simulink model "SVC"  (R2015b)
settings: Solver=VariableStepAuto  StartTime=0.0  StopTime=3  MaxStep=Ts  RelTol=1e-3
values from neighbouring files (symbols this model uses):
  f = 50    [ThreePhaseVSC_Code.m]
  FC_C = TSC_C    (= 3.3135e-06)    [ThreePhaseVSC_Code.m]
  FC_L = 122.3114e-3    (= 0.1223114)    [ThreePhaseVSC_Code.m]
  FC_R = 10    [ThreePhaseVSC_Code.m]
  L = XL/(2*2*pi*f)    (= 0.159154943092)    [ThreePhaseVSC_Code.m]
  TCR_L = 517.59e-3    (= 0.51759)    [ThreePhaseVSC_Code.m]
  TCR_R = 10    [ThreePhaseVSC_Code.m]
  Ts = 10e-6    (= 1e-05)    [ThreePhaseVSC_Code.m]
  TSC_C = 3.3135e-6    (= 3.3135e-06)    [ThreePhaseVSC_Code.m]
  TSC_L = 339.7539e-3    (= 0.3397539)    [ThreePhaseVSC_Code.m]
  TSC_R = 10    [ThreePhaseVSC_Code.m]
  Vr = 220e3    (= 220000)    [ThreePhaseVSC_Code.m]
  Vs = 220e3    (= 220000)    [ThreePhaseVSC_Code.m]
libraries: powerlib x56, powerlib_meascontrol x19, simulink x1
settings Model: Creator=Akshay Laturkar  LastModifiedBy=Sourabh Suri

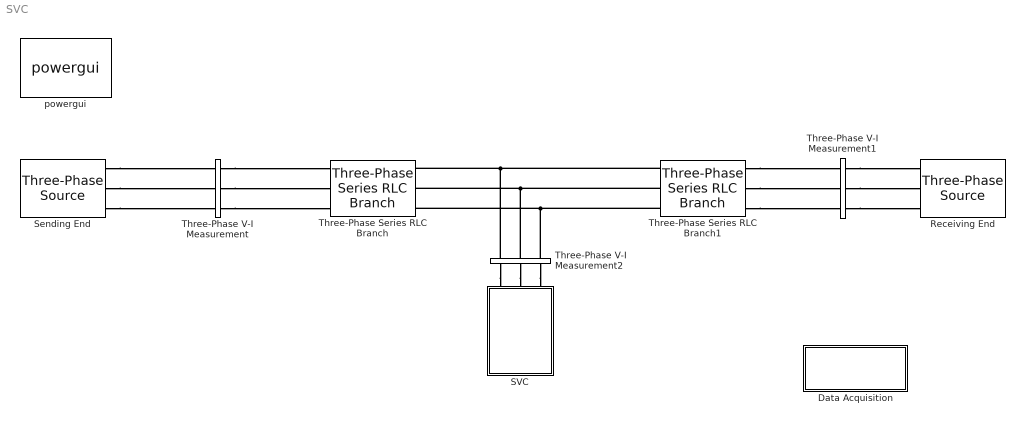
== system SVC ==
  Data Acquisition : Subsystem
  Receiving End : powerlib/Electrical Sources/Three-Phase Source  InternalConnection=Yg  VoltagePhases=off  Voltage=Vr  PhaseAngle=dr  Voltage_phases=[25e3 25e3 25e3]/sqrt(3)  PhaseAngles_phases=[0 -120 +120]  Frequency=f  NonIdealSource=off  SpecifyImpedance=off  Resistance=0.8929  Inductance=16.58e-3  ShortCircuitLevel=100e6  BaseVoltage=25e3  XRratio=7  BusType=swing  Pref=10e3  Qref=0  Prefabc=[10e3, 10e3, 10e3]  Qrefabc=[0, 0, 0]  Qmin=-inf  Qmax=inf
  SVC : Subsystem
  Sending End : powerlib/Electrical Sources/Three-Phase Source  InternalConnection=Yg  VoltagePhases=off  Voltage=Vs  PhaseAngle=ds  Voltage_phases=[25e3 25e3 25e3]/sqrt(3)  PhaseAngles_phases=[0 -120 +120]  Frequency=f  NonIdealSource=off  SpecifyImpedance=off  Resistance=0.8929  Inductance=16.58e-3  ShortCircuitLevel=100e6  BaseVoltage=25e3  XRratio=7  BusType=swing  Pref=10e3  Qref=0  Prefabc=[10e3, 10e3, 10e3]  Qrefabc=[0, 0, 0]  Qmin=-inf  Qmax=inf
  Three-Phase Series RLC Branch : powerlib/Elements/Three-Phase Series RLC Branch  LConnTagsString=A|B|C  RConnTagsString=A|B|C  BranchType=L  Resistance=1  Inductance=L  Capacitance=1e-6  Measurements=None
  Three-Phase Series RLC Branch1 : powerlib/Elements/Three-Phase Series RLC Branch  LConnTagsString=A|B|C  RConnTagsString=A|B|C  BranchType=L  Resistance=1  Inductance=L  Capacitance=1e-6  Measurements=None
  Three-Phase V-I Measurement : powerlib/Measurements/Three-Phase V-I Measurement  VoltageMeasurement=phase-to-phase  SetLabelV=on  LabelV=Vsabc  Vpu=off  VpuLL=on  CurrentMeasurement=yes  SetLabelI=on  LabelI=Isabc  Ipu=on  Pbase=Sbase  Vbase=Vn  OutputType=Complex  PhasorSimulation=off  PSBequivalent=0
  Three-Phase V-I Measurement1 : powerlib/Measurements/Three-Phase V-I Measurement  VoltageMeasurement=phase-to-phase  SetLabelV=on  LabelV=Vrabc  Vpu=off  VpuLL=on  CurrentMeasurement=yes  SetLabelI=on  LabelI=Irabc  Ipu=on  Pbase=Sbase  Vbase=Vn  OutputType=Complex  PhasorSimulation=off  PSBequivalent=0
  Three-Phase V-I Measurement2 : powerlib/Measurements/Three-Phase V-I Measurement  VoltageMeasurement=phase-to-phase  SetLabelV=on  LabelV=Vmabc  Vpu=off  VpuLL=on  CurrentMeasurement=yes  SetLabelI=on  LabelI=Imabc  Ipu=on  Pbase=Sbase  Vbase=Vn  OutputType=Complex  PhasorSimulation=off  PSBequivalent=0
  powergui : powerlib/powergui  Priority=1  SimulationMode=Discrete  SolverType=Backward Euler  SampleTime=Ts  frequency=60  SPID=off  DisableSnubberDevices=on  DisableRonSwitches=on  DisableVfSwitches=on  SwTol=0  DisplayEquations=off  Interpol=off  ExternalGateDelay=off  methode=off  Ts=10  FunctionMessages=off  echomessages=off  HookPort=off  EnableUseOfTLC=off  x0status=blocks  frequencyindice=0  Pbase=100e6  ErrMax=1e-4  Iterations=50  UnitsV=kV  UnitsW=MW  buscounter=0  RestoreLinks=warning  ResistiveCurrentMeasurement=off  Frange=[0:2:500]  Ylog=off  Xlog=on  ShowGrid=off  save=off  variable=ZData  structure=0  ZoomFFT=off  StartTime=0.0  cycles=1  DisplayStyle=1  fundamental=60  FreqAxis=off  MaxFrequency=1000  frequencyindicesteady=1  RmsSteady=1  display=off
  connections:
  Three-Phase V-I Measurement1/LConn1 -- Receiving End/RConn1
  Three-Phase V-I Measurement1/LConn2 -- Receiving End/RConn2
  Three-Phase V-I Measurement1/LConn3 -- Receiving End/RConn3
  Sending End/RConn1 -- Three-Phase V-I Measurement/LConn1
  Sending End/RConn2 -- Three-Phase V-I Measurement/LConn2
  Sending End/RConn3 -- Three-Phase V-I Measurement/LConn3
  Three-Phase Series RLC Branch1/LConn1 -- Three-Phase V-I Measurement1/RConn1
  Three-Phase Series RLC Branch1/LConn2 -- Three-Phase V-I Measurement1/RConn2
  Three-Phase Series RLC Branch1/LConn3 -- Three-Phase V-I Measurement1/RConn3
  Three-Phase V-I Measurement/RConn1 -- Three-Phase Series RLC Branch/LConn1
  Three-Phase V-I Measurement/RConn2 -- Three-Phase Series RLC Branch/LConn2
  Three-Phase V-I Measurement/RConn3 -- Three-Phase Series RLC Branch/LConn3
  Three-Phase Series RLC Branch1/RConn1 -- Three-Phase V-I Measurement2/RConn1 -- Three-Phase Series RLC Branch/RConn1
  Three-Phase Series RLC Branch1/RConn2 -- Three-Phase V-I Measurement2/RConn2 -- Three-Phase Series RLC Branch/RConn2
  Three-Phase Series RLC Branch1/RConn3 -- Three-Phase V-I Measurement2/RConn3 -- Three-Phase Series RLC Branch/RConn3
  Three-Phase V-I Measurement2/LConn1 -- SVC/LConn1
  Three-Phase V-I Measurement2/LConn2 -- SVC/LConn2
  Three-Phase V-I Measurement2/LConn3 -- SVC/LConn3

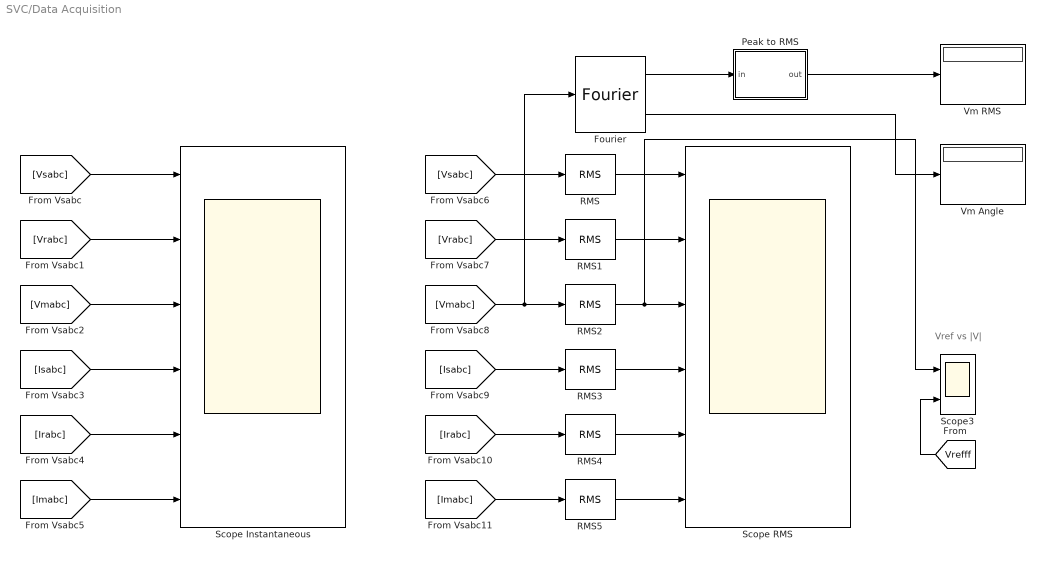
== system SVC/Data Acquisition ==
  note: Vref vs |V|
  Fourier : powerlib_meascontrol/Measurements/Fourier  Freq=f  n=1  InInit=[0, 0]  Ts=0
  Peak to RMS : MATLAB Function  TreatAsAtomicUnit=on
  RMS{,1..5} (6 alike) : powerlib_meascontrol/Measurements/RMS  TrueRMS=off  Freq=f  RMSInit=0  Ts=0
  Scope Instantaneous : Scope  NumInputPorts=6
  Scope RMS : Scope  NumInputPorts=6
  Scope3 : Scope  NumInputPorts=2
  Vm Angle : Display
      settings: Decimation=3
  Vm RMS : Display
      settings: Decimation=3
  wires:
  [Vsabc] -> Scope Instantaneous/1
  [Vrabc] -> Scope Instantaneous/2
  [Irabc] -> Scope Instantaneous/5
  [Imabc] -> Scope Instantaneous/6
  [Vmabc] -> Scope Instantaneous/3
  [Isabc] -> Scope Instantaneous/4
  RMS/1 -> Scope RMS/1
  [Vrabc] -> RMS1/1
  RMS1/1 -> Scope RMS/2
  [Vmabc] -> Fourier/1, RMS2/1
  [Isabc] -> RMS3/1
  RMS3/1 -> Scope RMS/4
  [Irabc] -> RMS4/1
  RMS4/1 -> Scope RMS/5
  [Imabc] -> RMS5/1
  RMS5/1 -> Scope RMS/6
  RMS2/1 -> Scope3/1, Scope RMS/3
  Fourier/2 -> Vm Angle/1
  [Vsabc] -> RMS/1
  Peak to RMS/1(out) -> Vm RMS/1
  Fourier/1 -> Peak to RMS/1(in)
  [Vrefff] -> Scope3/2

== system SVC/SVC ==
  FC TCR : Subsystem
  SVC Control : Subsystem
  TSC 1 : Subsystem
  TSC 2 : Subsystem
  A : PMIOPort  Port=1  Side=Left
  B : PMIOPort  Port=2  Side=Left
  C : PMIOPort  Port=3  Side=Left
  connections:
  A/RConn1 -- TSC 1/LConn1 -- TSC 2/RConn1 -- FC TCR/LConn1
  B/RConn1 -- TSC 1/LConn2 -- TSC 2/RConn2 -- FC TCR/LConn2
  C/RConn1 -- TSC 1/LConn3 -- TSC 2/RConn3 -- FC TCR/LConn3

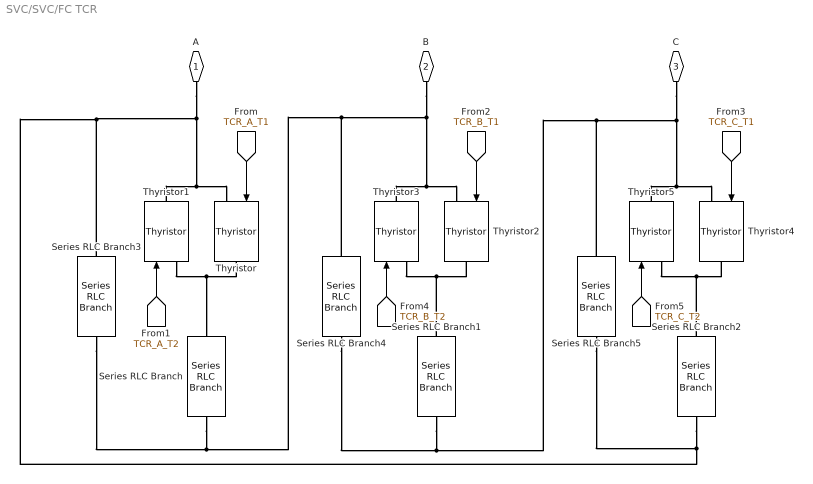
== system SVC/SVC/FC TCR ==
  Series RLC Branch : powerlib/Elements/Series RLC Branch  LConnTagsString=__new0  RConnTagsString=__new0  BranchType=RL  Resistance=TCR_R  Inductance=TCR_L  SetiL0=off  InitialCurrent=0  Capacitance=TSC_C  Setx0=off  InitialVoltage=0  Measurements=None
  Series RLC Branch1 : powerlib/Elements/Series RLC Branch  LConnTagsString=__new0  RConnTagsString=__new0  BranchType=RL  Resistance=TCR_R  Inductance=TCR_L  SetiL0=off  InitialCurrent=0  Capacitance=TSC_C  Setx0=off  InitialVoltage=0  Measurements=None
  Series RLC Branch2 : powerlib/Elements/Series RLC Branch  LConnTagsString=__new0  RConnTagsString=__new0  BranchType=RL  Resistance=TCR_R  Inductance=TCR_L  SetiL0=off  InitialCurrent=0  Capacitance=TSC_C  Setx0=off  InitialVoltage=0  Measurements=None
  Series RLC Branch3 : powerlib/Elements/Series RLC Branch  LConnTagsString=__new0  RConnTagsString=__new0  BranchType=RLC  Resistance=FC_R  Inductance=FC_L  SetiL0=off  InitialCurrent=0  Capacitance=FC_C  Setx0=off  InitialVoltage=0  Measurements=None
  Series RLC Branch4 : powerlib/Elements/Series RLC Branch  LConnTagsString=__new0  RConnTagsString=__new0  BranchType=RLC  Resistance=FC_R  Inductance=FC_L  SetiL0=off  InitialCurrent=0  Capacitance=FC_C  Setx0=off  InitialVoltage=0  Measurements=None
  Series RLC Branch5 : powerlib/Elements/Series RLC Branch  LConnTagsString=__new0  RConnTagsString=__new0  BranchType=RLC  Resistance=FC_R  Inductance=FC_L  SetiL0=off  InitialCurrent=0  Capacitance=FC_C  Setx0=off  InitialVoltage=0  Measurements=None
  Thyristor{,1..5} (6 alike) : powerlib/Power Electronics/Thyristor  Ron=Ron  Lon=0  Vf=Vf  IC=0  Rs=Snub_R  Cs=Snub_C  Measurements=off
  A : PMIOPort  Port=1  Side=Left
  B : PMIOPort  Port=2  Side=Left
  C : PMIOPort  Port=3  Side=Left
  wires:
  [TCR_A_T1] -> Thyristor/1
  [TCR_A_T2] -> Thyristor1/1
  [TCR_B_T1] -> Thyristor2/1
  [TCR_C_T1] -> Thyristor4/1
  [TCR_B_T2] -> Thyristor3/1
  [TCR_C_T2] -> Thyristor5/1
  connections:
  Thyristor5/LConn1 -- Series RLC Branch2/LConn1 -- Thyristor4/RConn1
  Thyristor3/LConn1 -- Series RLC Branch1/LConn1 -- Thyristor2/RConn1
  Thyristor/LConn1 -- A/RConn1 -- Series RLC Branch5/RConn1 -- Series RLC Branch2/RConn1 -- Series RLC Branch3/LConn1 -- Thyristor1/RConn1
  Thyristor3/RConn1 -- Thyristor2/LConn1 -- Series RLC Branch3/RConn1 -- Series RLC Branch/RConn1 -- Series RLC Branch4/LConn1 -- B/RConn1
  Thyristor5/RConn1 -- Series RLC Branch4/RConn1 -- Series RLC Branch1/RConn1 -- Series RLC Branch5/LConn1 -- C/RConn1 -- Thyristor4/LConn1
  Thyristor1/LConn1 -- Thyristor/RConn1 -- Series RLC Branch/LConn1

== system SVC/SVC/SVC Control ==
  Control Scheme 3phase : Subsystem
  Demux : Demux  Outputs=3
  Demux1 : Demux  Outputs=3
  Stair Generator2 : powerlib_meascontrol/Pulse & Signal Generators/Stair Generator  t=[0:.2:.8]  e=[0,.7,1.28,.7,1.28]  Ts=0
  Stair Generator3 : powerlib_meascontrol/Pulse & Signal Generators/Stair Generator  t=[0:.2:1.2]  e=[.7:0.1:1.3]  Ts=0
  TSC1 : Subsystem
  TSC2 : Subsystem
  tag scope: Vrefff=global
  wires:
  [TSC2_EN] -> TSC2/4(TSC2_EN)
  [TSC1_EN] -> TSC1/4(TSC1_EN)
  Demux/2 -> TSC1/2(Vm_B)
  Demux/1 -> TSC1/1(Vm_A)
  Demux/3 -> TSC1/3(Vm_C)
  [Vabc_TSC] -> Demux/1
  [Vabc_TSC2] -> Demux1/1
  Demux1/3 -> TSC2/3(Vm_C)
  Demux1/2 -> TSC2/2(Vm_B)
  Demux1/1 -> TSC2/1(Vm_A)
  Stair Generator3/1 -> [Vrefff], Control Scheme 3phase/1(Vdesired)

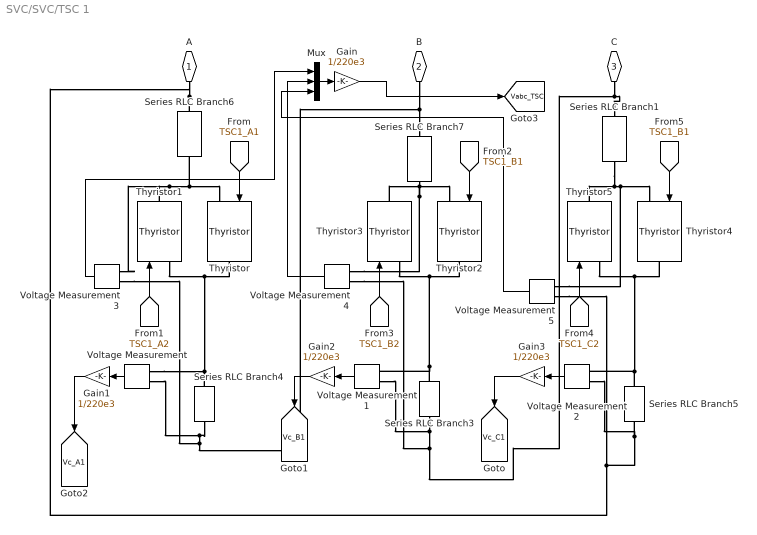
== system SVC/SVC/TSC 1 ==
  Gain{,1..3} (4 alike) : Gain  Gain=1/220e3
  Mux : Mux  Inputs=3
  Series RLC Branch1 : powerlib/Elements/Series RLC Branch  LConnTagsString=__new0  RConnTagsString=__new0  BranchType=RL  Resistance=TSC_R  Inductance=TSC_L  SetiL0=off  InitialCurrent=0  Capacitance=TSC_C  Setx0=off  InitialVoltage=0  Measurements=None
  Series RLC Branch3 : powerlib/Elements/Series RLC Branch  LConnTagsString=__new0  RConnTagsString=__new0  BranchType=C  Resistance=TSC_R  Inductance=TSC_L  SetiL0=off  InitialCurrent=0  Capacitance=TSC_C  Setx0=off  InitialVoltage=0  Measurements=None
  Series RLC Branch4 : powerlib/Elements/Series RLC Branch  LConnTagsString=__new0  RConnTagsString=__new0  BranchType=C  Resistance=TSC_R  Inductance=TSC_L  SetiL0=off  InitialCurrent=0  Capacitance=TSC_C  Setx0=off  InitialVoltage=0  Measurements=None
  Series RLC Branch5 : powerlib/Elements/Series RLC Branch  LConnTagsString=__new0  RConnTagsString=__new0  BranchType=C  Resistance=TSC_R  Inductance=TSC_L  SetiL0=off  InitialCurrent=0  Capacitance=TSC_C  Setx0=off  InitialVoltage=0  Measurements=None
  Series RLC Branch6 : powerlib/Elements/Series RLC Branch  LConnTagsString=__new0  RConnTagsString=__new0  BranchType=RL  Resistance=TSC_R  Inductance=TSC_L  SetiL0=off  InitialCurrent=0  Capacitance=TSC_C  Setx0=off  InitialVoltage=0  Measurements=None
  Series RLC Branch7 : powerlib/Elements/Series RLC Branch  LConnTagsString=__new0  RConnTagsString=__new0  BranchType=RL  Resistance=TSC_R  Inductance=TSC_L  SetiL0=off  InitialCurrent=0  Capacitance=TSC_C  Setx0=off  InitialVoltage=0  Measurements=None
  Thyristor{,1..5} (6 alike) : powerlib/Power Electronics/Thyristor  Ron=Ron  Lon=0  Vf=Vf  IC=0  Rs=Snub_R  Cs=Snub_C  Measurements=off
  Voltage Measurement{,1..5} (6 alike) : powerlib/Measurements/Voltage Measurement  PhasorSimulation=off  OutputType=Complex  PSBequivalent=0
  A : PMIOPort  Port=1  Side=Left
  B : PMIOPort  Port=2  Side=Left
  C : PMIOPort  Port=3  Side=Left
  tag scope: Vabc_TSC=global, Vc_A1=global, Vc_B1=global, Vc_C1=global
  wires:
  [TSC1_A1] -> Thyristor/1
  [TSC1_A2] -> Thyristor1/1
  [TSC1_B1] -> Thyristor2/1
  [TSC1_B2] -> Thyristor3/1
  [TSC1_C2] -> Thyristor5/1
  [TSC1_B1] -> Thyristor4/1
  Voltage Measurement2/1 -> Gain3/1
  Voltage Measurement1/1 -> Gain2/1
  Voltage Measurement/1 -> Gain1/1
  Voltage Measurement3/1 -> Mux/1
  Voltage Measurement4/1 -> Mux/2
  Voltage Measurement5/1 -> Mux/3
  Mux/1 -> Gain/1
  Gain/1 -> [Vabc_TSC]
  Gain1/1 -> [Vc_A1]
  Gain2/1 -> [Vc_B1]
  Gain3/1 -> [Vc_C1]
  connections:
  Thyristor5/RConn1 -- Series RLC Branch1/RConn1 -- Voltage Measurement5/LConn1 -- Thyristor4/LConn1
  Series RLC Branch3/LConn1 -- Thyristor3/LConn1 -- Thyristor2/RConn1 -- Voltage Measurement1/LConn1
  Thyristor3/RConn1 -- Series RLC Branch7/RConn1 -- Voltage Measurement4/LConn1 -- Thyristor2/LConn1
  Voltage Measurement2/LConn2 -- Series RLC Branch5/RConn1 -- Voltage Measurement5/LConn2 -- Series RLC Branch6/LConn1 -- A/RConn1
  Thyristor1/LConn1 -- Voltage Measurement/LConn1 -- Series RLC Branch4/LConn1 -- Thyristor/RConn1
  Thyristor5/LConn1 -- Series RLC Branch5/LConn1 -- Voltage Measurement2/LConn1 -- Thyristor4/RConn1
  Series RLC Branch6/RConn1 -- Voltage Measurement3/LConn1 -- Thyristor1/RConn1 -- Thyristor/LConn1
  Voltage Measurement3/LConn2 -- B/RConn1 -- Series RLC Branch7/LConn1 -- Voltage Measurement/LConn2 -- Series RLC Branch4/RConn1
  Voltage Measurement4/LConn2 -- C/RConn1 -- Series RLC Branch1/LConn1 -- Series RLC Branch3/RConn1 -- Voltage Measurement1/LConn2

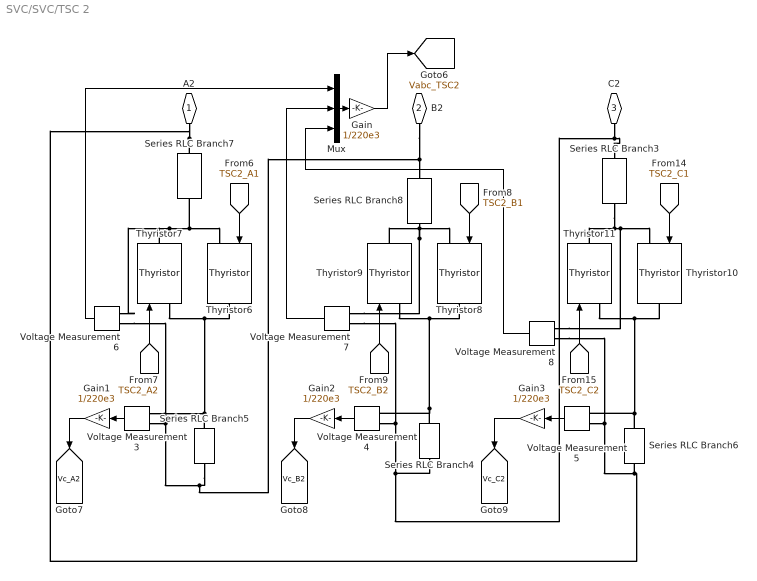
== system SVC/SVC/TSC 2 ==
  Gain{,1..3} (4 alike) : Gain  Gain=1/220e3
  Mux : Mux  Inputs=3
  Series RLC Branch3 : powerlib/Elements/Series RLC Branch  LConnTagsString=__new0  RConnTagsString=__new0  BranchType=RL  Resistance=TSC_R  Inductance=TSC_L  SetiL0=off  InitialCurrent=0  Capacitance=TSC_C  Setx0=off  InitialVoltage=0  Measurements=None
  Series RLC Branch4 : powerlib/Elements/Series RLC Branch  LConnTagsString=__new0  RConnTagsString=__new0  BranchType=C  Resistance=TSC_R  Inductance=TSC_L  SetiL0=off  InitialCurrent=0  Capacitance=TSC_C  Setx0=off  InitialVoltage=0  Measurements=None
  Series RLC Branch5 : powerlib/Elements/Series RLC Branch  LConnTagsString=__new0  RConnTagsString=__new0  BranchType=C  Resistance=TSC_R  Inductance=TSC_L  SetiL0=off  InitialCurrent=0  Capacitance=TSC_C  Setx0=off  InitialVoltage=0  Measurements=None
  Series RLC Branch6 : powerlib/Elements/Series RLC Branch  LConnTagsString=__new0  RConnTagsString=__new0  BranchType=C  Resistance=TSC_R  Inductance=TSC_L  SetiL0=off  InitialCurrent=0  Capacitance=TSC_C  Setx0=off  InitialVoltage=0  Measurements=None
  Series RLC Branch7 : powerlib/Elements/Series RLC Branch  LConnTagsString=__new0  RConnTagsString=__new0  BranchType=RL  Resistance=TSC_R  Inductance=TSC_L  SetiL0=off  InitialCurrent=0  Capacitance=TSC_C  Setx0=off  InitialVoltage=0  Measurements=None
  Series RLC Branch8 : powerlib/Elements/Series RLC Branch  LConnTagsString=__new0  RConnTagsString=__new0  BranchType=RL  Resistance=TSC_R  Inductance=TSC_L  SetiL0=off  InitialCurrent=0  Capacitance=TSC_C  Setx0=off  InitialVoltage=0  Measurements=None
  Thyristor{6..11} (6 alike) : powerlib/Power Electronics/Thyristor  Ron=Ron  Lon=0  Vf=Vf  IC=0  Rs=Snub_R  Cs=Snub_C  Measurements=off
  Voltage Measurement{3..8} (6 alike) : powerlib/Measurements/Voltage Measurement  PhasorSimulation=off  OutputType=Complex  PSBequivalent=0
  A2 : PMIOPort  Port=1  Side=Right
  B2 : PMIOPort  Port=2  Side=Right
  C2 : PMIOPort  Port=3  Side=Right
  tag scope: Vabc_TSC2=global, Vc_A2=global, Vc_B2=global, Vc_C2=global
  wires:
  [TSC2_A1] -> Thyristor6/1
  [TSC2_A2] -> Thyristor7/1
  [TSC2_B1] -> Thyristor8/1
  [TSC2_B2] -> Thyristor9/1
  [TSC2_C2] -> Thyristor11/1
  [TSC2_C1] -> Thyristor10/1
  Voltage Measurement5/1 -> Gain3/1
  Voltage Measurement4/1 -> Gain2/1
  Voltage Measurement3/1 -> Gain1/1
  Voltage Measurement6/1 -> Mux/1
  Voltage Measurement7/1 -> Mux/2
  Voltage Measurement8/1 -> Mux/3
  Mux/1 -> Gain/1
  Gain/1 -> [Vabc_TSC2]
  Gain1/1 -> [Vc_A2]
  Gain2/1 -> [Vc_B2]
  Gain3/1 -> [Vc_C2]
  connections:
  Thyristor10/LConn1 -- Voltage Measurement8/LConn1 -- Series RLC Branch3/RConn1 -- Thyristor11/RConn1
  Series RLC Branch4/LConn1 -- Thyristor9/LConn1 -- Thyristor8/RConn1 -- Voltage Measurement4/LConn1
  Thyristor8/LConn1 -- Series RLC Branch8/RConn1 -- Voltage Measurement7/LConn1 -- Thyristor9/RConn1
  A2/RConn1 -- Series RLC Branch7/LConn1 -- Voltage Measurement5/LConn2 -- Voltage Measurement8/LConn2 -- Series RLC Branch6/RConn1
  Thyristor6/RConn1 -- Voltage Measurement3/LConn1 -- Series RLC Branch5/LConn1 -- Thyristor7/LConn1
  Thyristor10/RConn1 -- Series RLC Branch6/LConn1 -- Voltage Measurement5/LConn1 -- Thyristor11/LConn1
  Series RLC Branch7/RConn1 -- Voltage Measurement6/LConn1 -- Thyristor7/RConn1 -- Thyristor6/LConn1
  B2/RConn1 -- Voltage Measurement6/LConn2 -- Voltage Measurement3/LConn2 -- Series RLC Branch5/RConn1 -- Series RLC Branch8/LConn1
  Voltage Measurement4/LConn2 -- Series RLC Branch4/RConn1 -- C2/RConn1 -- Series RLC Branch3/LConn1 -- Voltage Measurement7/LConn2

== system SVC/SVC/SVC Control/Control Scheme 3phase ==
  Vdesired : Inport
  Demux : Demux  Outputs=3
  Display8 : Display
  MATLAB Function2 : MATLAB Function  TreatAsAtomicUnit=on
  Mux : Mux
  PLL : powerlib_meascontrol/PLL/PLL  Fmin=45  Par_Init=[0, 50.1]  ParK=[180, 3200, 1]  TcD=1e-4  MaxRateChangeFreq=12  FilterCutOffFreq=25  Ts=0  AGC=on
  PLL1 : powerlib_meascontrol/PLL/PLL  Fmin=45  Par_Init=[0, 50.1]  ParK=[180, 3200, 1]  TcD=1e-4  MaxRateChangeFreq=12  FilterCutOffFreq=25  Ts=0  AGC=on
  PLL2 : powerlib_meascontrol/PLL/PLL  Fmin=45  Par_Init=[0, 50.1]  ParK=[180, 3200, 1]  TcD=1e-4  MaxRateChangeFreq=12  FilterCutOffFreq=25  Ts=0  AGC=on
  Pulse Generator3 : Subsystem
  Subsystem : Subsystem
  Terminator : Terminator
  Terminator1 : Terminator
  Terminator2 : Terminator
  tag scope: TSC1_EN=global, TSC2_EN=global
  wires:
  MATLAB Function2/3(TSC1_EN) -> [TSC1_EN], Mux/3
  MATLAB Function2/4(TSC2_EN) -> [TSC2_EN], Mux/4
  Vdesired/1 -> MATLAB Function2/1(Vdesired)
  Mux/1 -> Display8/1
  MATLAB Function2/2(FCTCR_EN) -> Pulse Generator3/5(Enable), Mux/2
  PLL/2 -> MATLAB Function2/2(wta)
  MATLAB Function2/6(wt_half_b) -> Pulse Generator3/2(wt_half 1)
  PLL1/2 -> MATLAB Function2/3(wtb)
  Demux/1 -> PLL/1
  Demux/2 -> PLL1/1
  Demux/3 -> PLL2/1
  [Vmabc] -> Demux/1
  PLL1/1 -> Terminator1/1
  PLL2/1 -> Terminator2/1
  PLL2/2 -> MATLAB Function2/4(wtc)
  PLL/1 -> Terminator/1
  MATLAB Function2/1(triggerlevel) -> Pulse Generator3/4("TriggerLevel "), Mux/1
  MATLAB Function2/7(wt_half_c) -> Pulse Generator3/3(wt_half 2)
  MATLAB Function2/5(wt_half_a) -> Pulse Generator3/1("wt_half ")

== system SVC/SVC/SVC Control/TSC1 ==
  Vm_A : Inport
  Vm_B : Inport  Port=2
  Vm_C : Inport  Port=3
  TSC1_EN : Inport  Port=4
  TSC_Control/phase a : Subsystem
  TSC_Control/phase b : Subsystem
  TSC_Control/phase c : Subsystem
  tag scope: TSC1_A1=global, TSC1_A2=global, TSC1_B1=global, TSC1_B2=global, TSC1_C1=global, TSC1_C2=global
  wires:
  Vm_A/1 -> TSC_Control/phase a/1(In1)
  Vm_B/1 -> TSC_Control/phase b/1(In1)
  Vm_C/1 -> TSC_Control/phase c/1(In1)
  TSC1_EN/1 -> TSC_Control/phase c/2(In2), TSC_Control/phase b/2(In2), TSC_Control/phase a/2(In2)
  TSC_Control/phase a/1(T1) -> [TSC1_A1]
  TSC_Control/phase a/2(T2) -> [TSC1_A2]
  TSC_Control/phase b/1(T1) -> [TSC1_B1]
  TSC_Control/phase b/2(T2) -> [TSC1_B2]
  TSC_Control/phase c/1(T1) -> [TSC1_C1]
  TSC_Control/phase c/2(T2) -> [TSC1_C2]

== system SVC/SVC/SVC Control/TSC2 ==
  Vm_A : Inport
  Vm_B : Inport  Port=2
  Vm_C : Inport  Port=3
  TSC2_EN : Inport  Port=4
  TSC_Control/phase a : Subsystem
  TSC_Control/phase b : Subsystem
  TSC_Control/phase c : Subsystem
  tag scope: TSC2_A1=global, TSC2_A2=global, TSC2_B1=global, TSC2_B2=global, TSC2_C1=global, TSC2_C2=global
  wires:
  TSC2_EN/1 -> TSC_Control/phase a/2(In2), TSC_Control/phase b/2(In2), TSC_Control/phase c/2(In2)
  Vm_C/1 -> TSC_Control/phase c/1(In1)
  Vm_B/1 -> TSC_Control/phase b/1(In1)
  Vm_A/1 -> TSC_Control/phase a/1(In1)
  TSC_Control/phase a/1(T1) -> [TSC2_A1]
  TSC_Control/phase a/2(T2) -> [TSC2_A2]
  TSC_Control/phase b/1(T1) -> [TSC2_B1]
  TSC_Control/phase b/2(T2) -> [TSC2_B2]
  TSC_Control/phase c/1(T1) -> [TSC2_C1]
  TSC_Control/phase c/2(T2) -> [TSC2_C2]

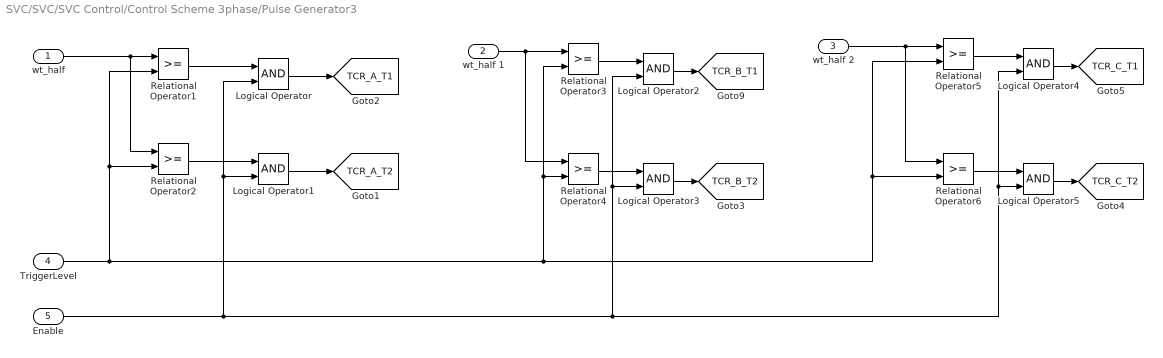
== system SVC/SVC/SVC Control/Control Scheme 3phase/Pulse Generator3 ==
  "wt_half " : Inport
  wt_half 1 : Inport  Port=2
  wt_half 2 : Inport  Port=3
  "TriggerLevel " : Inport  Port=4
  Enable : Inport  Port=5
  Logical Operator{,1..5} (6 alike) : Logic  AllPortsSameDT=off  OutDataTypeStr=boolean
  Relational Operator{1..6} (6 alike) : RelationalOperator  OutDataTypeStr=boolean
  tag scope: TCR_A_T1=global, TCR_A_T2=global, TCR_B_T1=global, TCR_B_T2=global, TCR_C_T1=global, TCR_C_T2=global
  wires:
  "TriggerLevel "/1 -> Relational Operator2/2, Relational Operator1/2, Relational Operator5/2, Relational Operator6/2, Relational Operator4/2, Relational Operator3/2
  "wt_half "/1 -> Relational Operator2/1, Relational Operator1/1
  Relational Operator1/1 -> Logical Operator/1
  Logical Operator/1 -> [TCR_A_T1]
  Logical Operator1/1 -> [TCR_A_T2]
  Relational Operator2/1 -> Logical Operator1/1
  Enable/1 -> Logical Operator4/2, Logical Operator5/2, Logical Operator2/2, Logical Operator3/2, Logical Operator/2, Logical Operator1/2
  wt_half 1/1 -> Relational Operator4/1, Relational Operator3/1
  wt_half 2/1 -> Relational Operator6/1, Relational Operator5/1
  Relational Operator3/1 -> Logical Operator2/1
  Relational Operator4/1 -> Logical Operator3/1
  Logical Operator2/1 -> [TCR_B_T1]
  Logical Operator3/1 -> [TCR_B_T2]
  Relational Operator5/1 -> Logical Operator4/1
  Relational Operator6/1 -> Logical Operator5/1
  Logical Operator4/1 -> [TCR_C_T1]
  Logical Operator5/1 -> [TCR_C_T2]

== system SVC/SVC/SVC Control/Control Scheme 3phase/Subsystem ==
  In1 : Inport
  Constant : Constant  Value=264.31
  Divide : Product  Inputs=*/
  PID Controller1 : simulink/Continuous/PID Controller  Controller=PI  TimeDomain=Continuous-time  SampleTime=-1  IntegratorMethod=Forward Euler  FilterMethod=Forward Euler  Form=Parallel  UseFilter=on  ControllerParametersSource=internal  P=.0075  I=.002  D=0  N=100  InitialConditionSource=internal  InitialConditionForIntegrator=0  InitialConditionForFilter=0  ExternalReset=none  LimitOutput=off  UpperSaturationLimit=inf  LowerSaturationLimit=-inf  LinearizeAsGain=on  AntiWindupMode=none  Kb=1  TrackingMode=off  Kt=1  PParamMin=[]  PParamMax=[]  IParamMin=[]  IParamMax=[]  DParamMin=[]  DParamMax=[]  NParamMin=[]  NParamMax=[]  KbParamMin=[]  KbParamMax=[]  KtParamMin=[]  KtParamMax=[]  POutMin=[]  POutMax=[]  IOutMin=[]  IOutMax=[]  DOutMin=[]  DOutMax=[]  NOutMin=[]  NOutMax=[]  KbOutMin=[]  KbOutMax=[]  KtOutMin=[]  KtOutMax=[]  IntegratorOutMin=[]  IntegratorOutMax=[]  FilterOutMin=[]  FilterOutMax=[]  SumOutMin=[]  SumOutMax=[]  SumI1OutMin=[]  SumI1OutMax=[]  SumI2OutMin=[]  SumI2OutMax=[]  SumI3OutMin=[]  SumI3OutMax=[]  SumDOutMin=[]  SumDOutMax=[]  SaturationOutMin=[]  SaturationOutMax=[]  IntegratorContinuousStateAttributes=''  IntegratorStateMustResolveToSignalObject=off  IntegratorRTWStateStorageClass=Auto  FilterContinuousStateAttributes=''  FilterStateMustResolveToSignalObject=off  FilterRTWStateStorageClass=Auto  DifferentiatorICPrevScaledInput=0  DifferentiatorOutMin=[]  DifferentiatorOutMax=[]
  RMS : powerlib_meascontrol/Measurements/RMS  TrueRMS=off  Freq=f  RMSInit=0  Ts=0
  Sum : Sum  Inputs=+-
  Out1 : Outport
  wires:
  [IL] -> RMS/1
  Constant/1 -> Divide/2
  Divide/1 -> Sum/2
  PID Controller1/1 -> Out1/1
  Sum/1 -> PID Controller1/1
  RMS/1 -> Divide/1
  In1/1 -> Sum/1

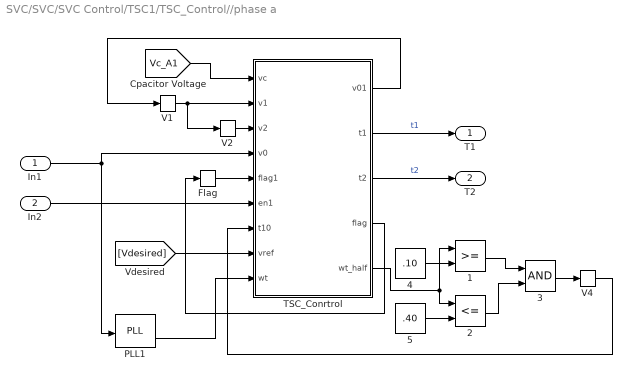
== system SVC/SVC/SVC Control/TSC1/TSC_Control//phase a ==
  In1 : Inport
  In2 : Inport  Port=2
  1 : RelationalOperator  OutDataTypeStr=boolean
  2 : RelationalOperator  Operator=<=  OutDataTypeStr=boolean
  "3 " : Logic  AllPortsSameDT=off  OutDataTypeStr=boolean
  4 : Constant  Value=.10
  5 : Constant  Value=.40
  Flag : Memory  InheritSampleTime=on  LinearizeMemory=on  LinearizeAsDelay=on
  PLL1 : powerlib_meascontrol/PLL/PLL  Fmin=45  Par_Init=[0, 50.1]  ParK=[180, 3200, 1]  TcD=1e-4  MaxRateChangeFreq=12  FilterCutOffFreq=25  Ts=0  AGC=on
  TSC_Conrtrol : MATLAB Function  TreatAsAtomicUnit=on
  V1 : Memory  InheritSampleTime=on  LinearizeMemory=on  LinearizeAsDelay=on
  V2 : Memory  InheritSampleTime=on  LinearizeMemory=on  LinearizeAsDelay=on
  V4 : Memory  InheritSampleTime=on  LinearizeMemory=on  LinearizeAsDelay=on
  T1 : Outport
  T2 : Outport  Port=2
  wires:
  TSC_Conrtrol/2(t1) -> T1/1  "t1"
  V1/1 -> TSC_Conrtrol/2(v1), V2/1
  TSC_Conrtrol/1(v01) -> V1/1
  4/1 -> 1/2
  PLL1/2 -> TSC_Conrtrol/9(wt)
  [Vdesired] -> TSC_Conrtrol/8(vref)
  "3 "/1 -> V4/1
  In1/1 -> TSC_Conrtrol/4(v0), PLL1/1
  In2/1 -> TSC_Conrtrol/6(en1)
  2/1 -> "3 "/2
  5/1 -> 2/2
  1/1 -> "3 "/1
  [Vc_A1] -> TSC_Conrtrol/1(vc)
  V2/1 -> TSC_Conrtrol/3(v2)
  TSC_Conrtrol/4(flag) -> Flag/1
  Flag/1 -> TSC_Conrtrol/5(flag1)
  TSC_Conrtrol/3(t2) -> T2/1  "t2"
  TSC_Conrtrol/5(wt_half) -> 1/1, 2/1
  V4/1 -> TSC_Conrtrol/7(t10)

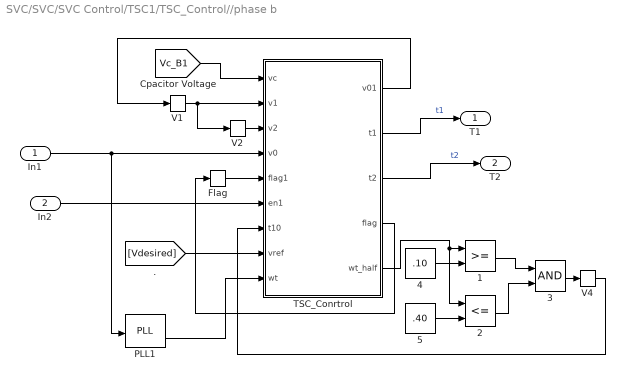
== system SVC/SVC/SVC Control/TSC1/TSC_Control//phase b ==
  In1 : Inport
  In2 : Inport  Port=2
  1 : RelationalOperator  OutDataTypeStr=boolean
  2 : RelationalOperator  Operator=<=  OutDataTypeStr=boolean
  "3 " : Logic  AllPortsSameDT=off  OutDataTypeStr=boolean
  4 : Constant  Value=.10
  5 : Constant  Value=.40
  Flag : Memory  InheritSampleTime=on  LinearizeMemory=on  LinearizeAsDelay=on
  PLL1 : powerlib_meascontrol/PLL/PLL  Fmin=45  Par_Init=[0, 50.1]  ParK=[180, 3200, 1]  TcD=1e-4  MaxRateChangeFreq=12  FilterCutOffFreq=25  Ts=0  AGC=on
  TSC_Conrtrol : MATLAB Function  TreatAsAtomicUnit=on
  V1 : Memory  InheritSampleTime=on  LinearizeMemory=on  LinearizeAsDelay=on
  V2 : Memory  InheritSampleTime=on  LinearizeMemory=on  LinearizeAsDelay=on
  V4 : Memory  InheritSampleTime=on  LinearizeMemory=on  LinearizeAsDelay=on
  T1 : Outport
  T2 : Outport  Port=2
  wires:
  TSC_Conrtrol/2(t1) -> T1/1  "t1"
  V1/1 -> TSC_Conrtrol/2(v1), V2/1
  TSC_Conrtrol/1(v01) -> V1/1
  4/1 -> 1/2
  PLL1/2 -> TSC_Conrtrol/9(wt)
  [Vdesired] -> TSC_Conrtrol/8(vref)
  "3 "/1 -> V4/1
  In1/1 -> PLL1/1, TSC_Conrtrol/4(v0)
  In2/1 -> TSC_Conrtrol/6(en1)
  2/1 -> "3 "/2
  5/1 -> 2/2
  1/1 -> "3 "/1
  [Vc_B1] -> TSC_Conrtrol/1(vc)
  V2/1 -> TSC_Conrtrol/3(v2)
  TSC_Conrtrol/4(flag) -> Flag/1
  Flag/1 -> TSC_Conrtrol/5(flag1)
  TSC_Conrtrol/3(t2) -> T2/1  "t2"
  TSC_Conrtrol/5(wt_half) -> 2/1, 1/1
  V4/1 -> TSC_Conrtrol/7(t10)

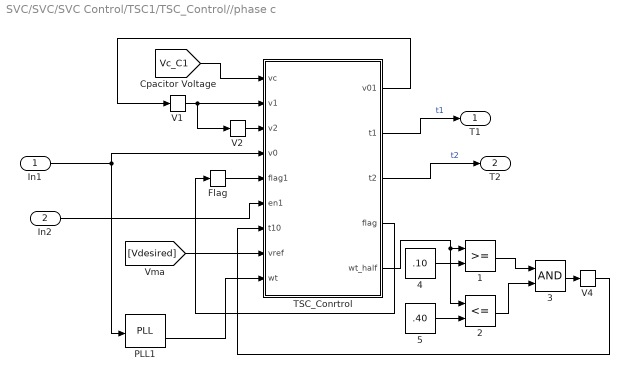
== system SVC/SVC/SVC Control/TSC1/TSC_Control//phase c ==
  In1 : Inport
  In2 : Inport  Port=2
  1 : RelationalOperator  OutDataTypeStr=boolean
  2 : RelationalOperator  Operator=<=  OutDataTypeStr=boolean
  "3 " : Logic  AllPortsSameDT=off  OutDataTypeStr=boolean
  4 : Constant  Value=.10
  5 : Constant  Value=.40
  Flag : Memory  InheritSampleTime=on  LinearizeMemory=on  LinearizeAsDelay=on
  PLL1 : powerlib_meascontrol/PLL/PLL  Fmin=45  Par_Init=[0, 50.1]  ParK=[180, 3200, 1]  TcD=1e-4  MaxRateChangeFreq=12  FilterCutOffFreq=25  Ts=0  AGC=on
  TSC_Conrtrol : MATLAB Function  TreatAsAtomicUnit=on
  V1 : Memory  InheritSampleTime=on  LinearizeMemory=on  LinearizeAsDelay=on
  V2 : Memory  InheritSampleTime=on  LinearizeMemory=on  LinearizeAsDelay=on
  V4 : Memory  InheritSampleTime=on  LinearizeMemory=on  LinearizeAsDelay=on
  T1 : Outport
  T2 : Outport  Port=2
  wires:
  TSC_Conrtrol/2(t1) -> T1/1  "t1"
  V1/1 -> TSC_Conrtrol/2(v1), V2/1
  TSC_Conrtrol/1(v01) -> V1/1
  4/1 -> 1/2
  PLL1/2 -> TSC_Conrtrol/9(wt)
  [Vdesired] -> TSC_Conrtrol/8(vref)
  "3 "/1 -> V4/1
  In1/1 -> TSC_Conrtrol/4(v0), PLL1/1
  In2/1 -> TSC_Conrtrol/6(en1)
  2/1 -> "3 "/2
  5/1 -> 2/2
  1/1 -> "3 "/1
  [Vc_C1] -> TSC_Conrtrol/1(vc)
  V2/1 -> TSC_Conrtrol/3(v2)
  TSC_Conrtrol/4(flag) -> Flag/1
  Flag/1 -> TSC_Conrtrol/5(flag1)
  TSC_Conrtrol/3(t2) -> T2/1  "t2"
  TSC_Conrtrol/5(wt_half) -> 2/1, 1/1
  V4/1 -> TSC_Conrtrol/7(t10)

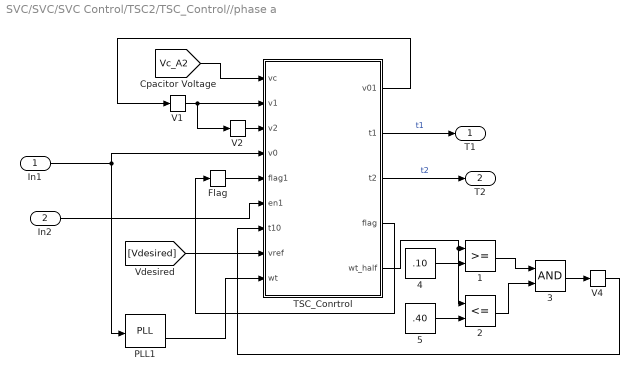
== system SVC/SVC/SVC Control/TSC2/TSC_Control//phase a ==
  In1 : Inport
  In2 : Inport  Port=2
  1 : RelationalOperator  OutDataTypeStr=boolean
  2 : RelationalOperator  Operator=<=  OutDataTypeStr=boolean
  "3 " : Logic  AllPortsSameDT=off  OutDataTypeStr=boolean
  4 : Constant  Value=.10
  5 : Constant  Value=.40
  Flag : Memory  InheritSampleTime=on  LinearizeMemory=on  LinearizeAsDelay=on
  PLL1 : powerlib_meascontrol/PLL/PLL  Fmin=45  Par_Init=[0, 50.1]  ParK=[180, 3200, 1]  TcD=1e-4  MaxRateChangeFreq=12  FilterCutOffFreq=25  Ts=0  AGC=on
  TSC_Conrtrol : MATLAB Function  TreatAsAtomicUnit=on
  V1 : Memory  InheritSampleTime=on  LinearizeMemory=on  LinearizeAsDelay=on
  V2 : Memory  InheritSampleTime=on  LinearizeMemory=on  LinearizeAsDelay=on
  V4 : Memory  InheritSampleTime=on  LinearizeMemory=on  LinearizeAsDelay=on
  T1 : Outport
  T2 : Outport  Port=2
  wires:
  TSC_Conrtrol/3(t2) -> T2/1  "t2"
  Flag/1 -> TSC_Conrtrol/5(flag1)
  TSC_Conrtrol/4(flag) -> Flag/1
  V2/1 -> TSC_Conrtrol/3(v2)
  [Vc_A2] -> TSC_Conrtrol/1(vc)
  1/1 -> "3 "/1
  5/1 -> 2/2
  2/1 -> "3 "/2
  In2/1 -> TSC_Conrtrol/6(en1)
  In1/1 -> PLL1/1, TSC_Conrtrol/4(v0)
  "3 "/1 -> V4/1
  [Vdesired] -> TSC_Conrtrol/8(vref)
  PLL1/2 -> TSC_Conrtrol/9(wt)
  4/1 -> 1/2
  TSC_Conrtrol/1(v01) -> V1/1
  V1/1 -> V2/1, TSC_Conrtrol/2(v1)
  TSC_Conrtrol/2(t1) -> T1/1  "t1"
  TSC_Conrtrol/5(wt_half) -> 2/1, 1/1
  V4/1 -> TSC_Conrtrol/7(t10)

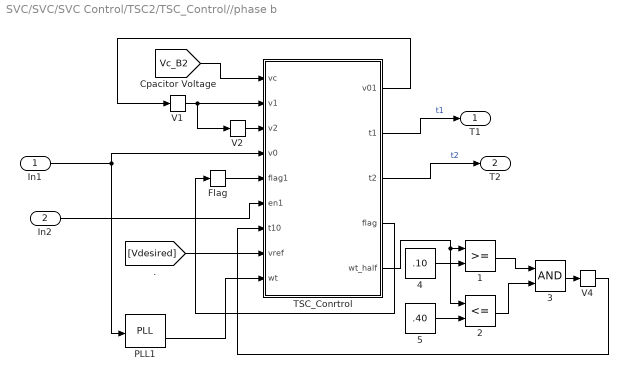
== system SVC/SVC/SVC Control/TSC2/TSC_Control//phase b ==
  In1 : Inport
  In2 : Inport  Port=2
  1 : RelationalOperator  OutDataTypeStr=boolean
  2 : RelationalOperator  Operator=<=  OutDataTypeStr=boolean
  "3 " : Logic  AllPortsSameDT=off  OutDataTypeStr=boolean
  4 : Constant  Value=.10
  5 : Constant  Value=.40
  Flag : Memory  InheritSampleTime=on  LinearizeMemory=on  LinearizeAsDelay=on
  PLL1 : powerlib_meascontrol/PLL/PLL  Fmin=45  Par_Init=[0, 50.1]  ParK=[180, 3200, 1]  TcD=1e-4  MaxRateChangeFreq=12  FilterCutOffFreq=25  Ts=0  AGC=on
  TSC_Conrtrol : MATLAB Function  TreatAsAtomicUnit=on
  V1 : Memory  InheritSampleTime=on  LinearizeMemory=on  LinearizeAsDelay=on
  V2 : Memory  InheritSampleTime=on  LinearizeMemory=on  LinearizeAsDelay=on
  V4 : Memory  InheritSampleTime=on  LinearizeMemory=on  LinearizeAsDelay=on
  T1 : Outport
  T2 : Outport  Port=2
  wires:
  TSC_Conrtrol/3(t2) -> T2/1  "t2"
  Flag/1 -> TSC_Conrtrol/5(flag1)
  TSC_Conrtrol/4(flag) -> Flag/1
  V2/1 -> TSC_Conrtrol/3(v2)
  [Vc_B2] -> TSC_Conrtrol/1(vc)
  1/1 -> "3 "/1
  5/1 -> 2/2
  2/1 -> "3 "/2
  In2/1 -> TSC_Conrtrol/6(en1)
  In1/1 -> PLL1/1, TSC_Conrtrol/4(v0)
  "3 "/1 -> V4/1
  [Vdesired] -> TSC_Conrtrol/8(vref)
  PLL1/2 -> TSC_Conrtrol/9(wt)
  4/1 -> 1/2
  TSC_Conrtrol/1(v01) -> V1/1
  V1/1 -> V2/1, TSC_Conrtrol/2(v1)
  TSC_Conrtrol/2(t1) -> T1/1  "t1"
  TSC_Conrtrol/5(wt_half) -> 2/1, 1/1
  V4/1 -> TSC_Conrtrol/7(t10)

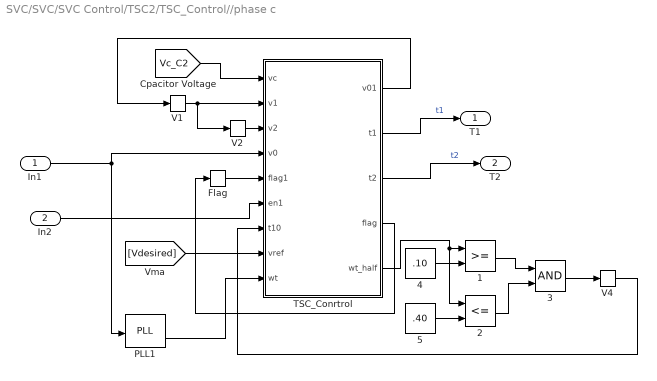
== system SVC/SVC/SVC Control/TSC2/TSC_Control//phase c ==
  In1 : Inport
  In2 : Inport  Port=2
  1 : RelationalOperator  OutDataTypeStr=boolean
  2 : RelationalOperator  Operator=<=  OutDataTypeStr=boolean
  "3 " : Logic  AllPortsSameDT=off  OutDataTypeStr=boolean
  4 : Constant  Value=.10
  5 : Constant  Value=.40
  Flag : Memory  InheritSampleTime=on  LinearizeMemory=on  LinearizeAsDelay=on
  PLL1 : powerlib_meascontrol/PLL/PLL  Fmin=45  Par_Init=[0, 50.1]  ParK=[180, 3200, 1]  TcD=1e-4  MaxRateChangeFreq=12  FilterCutOffFreq=25  Ts=0  AGC=on
  TSC_Conrtrol : MATLAB Function  TreatAsAtomicUnit=on
  V1 : Memory  InheritSampleTime=on  LinearizeMemory=on  LinearizeAsDelay=on
  V2 : Memory  InheritSampleTime=on  LinearizeMemory=on  LinearizeAsDelay=on
  V4 : Memory  InheritSampleTime=on  LinearizeMemory=on  LinearizeAsDelay=on
  T1 : Outport
  T2 : Outport  Port=2
  wires:
  TSC_Conrtrol/3(t2) -> T2/1  "t2"
  Flag/1 -> TSC_Conrtrol/5(flag1)
  TSC_Conrtrol/4(flag) -> Flag/1
  V2/1 -> TSC_Conrtrol/3(v2)
  [Vc_C2] -> TSC_Conrtrol/1(vc)
  1/1 -> "3 "/1
  5/1 -> 2/2
  2/1 -> "3 "/2
  In2/1 -> TSC_Conrtrol/6(en1)
  In1/1 -> PLL1/1, TSC_Conrtrol/4(v0)
  "3 "/1 -> V4/1
  [Vdesired] -> TSC_Conrtrol/8(vref)
  PLL1/2 -> TSC_Conrtrol/9(wt)
  4/1 -> 1/2
  TSC_Conrtrol/1(v01) -> V1/1
  V1/1 -> V2/1, TSC_Conrtrol/2(v1)
  TSC_Conrtrol/2(t1) -> T1/1  "t1"
  TSC_Conrtrol/5(wt_half) -> 2/1, 1/1
  V4/1 -> TSC_Conrtrol/7(t10)

== matlab function SVC/Data Acquisition/Peak to RMS ==
  data: in input; out output
function out = fcn(in)
% converts peak values to RMS values

out = in/sqrt(2);

== matlab function SVC/SVC Control/TSC1/TSC_Control//phase a/TSC_Conrtrol ==
  data: v01 output; t1 output; t2 output; vc input; v1 input; v2 input; v0 input; flag output; flag1 input; en1 input; t10 input; vref input; wt input; wt_half output
function [v01,t1,t2,flag,wt_half] = TSC_control(vc,v1,v2,v0,flag1,en1,t10,vref,wt)
wt=wt/(2*pi);
if(wt>=0.5)
    wt_half = wt - 0.5;
else
    wt_half = wt;
end
flag =flag1;
v01=v0;
     t1=0;
     t2=0;

if en1==1
  
   if flag>1 
             

                if (t10==1)
                t1=1; t2=1;

                else 
                    t1=0;t2=0;
                end
         if vref>1.29
            t1=1;t2=1;
         end 


   elseif flag<1
        t1=0;
        t2=0;
        if abs(vc)< 1e-5 && abs(v0)<1e-2
             t2=1;
              t1=1;
                
                    flag=flag+.005;
        end
        if vc>=0 && v0>0
            if abs(v0-vc)<1e-3 || (v1 > v2 && v1>v0 && vc>v1)
                    t2=1;
                    t1=1;
                
                    flag=flag+.005;
            end
        end
        if vc<=0 && v0<0
            if abs(v0-vc)<1e-3|| (v1<v2 && v1<v0 && vc<v1)
                    t1=1;
                    t2=1;
                    flag=flag+.005;
            end
        end
  end
    
end
    
if en1==0
    flag=0;
end

== matlab function SVC/SVC Control/Control Scheme 3phase/MATLAB Function2 ==
  data: Vdesired input; triggerlevel output; FCTCR_EN output; TSC1_EN output; TSC2_EN output; wta input; wt_half_a output; wtb input; wtc input; wt_half_b output; wt_half_c output
function [triggerlevel,FCTCR_EN,TSC1_EN,TSC2_EN,wt_half_a,wt_half_b,wt_half_c] = fcn(Vdesired,wta,wtb,wtc)
mul=1;
%#Frequency Division Code
    wta=wta/(2*pi);
    wtc=wtc/(2*pi);
    wtb=wtb/(2*pi);
        if(wta>=0.5)
            wt_half_a = mul*(wta - 0.5) ;
        else
            wt_half_a = mul*wta;
        end
        
        if(wtb>=0.5)
            wt_half_b = mul*(wtb - 0.5);
        else
            wt_half_b = mul*wtb;
        end
        
                if(wtc>=0.5)
            wt_half_c = mul*(wtc - 0.5);
        else
            wt_half_c = mul*(wtc);
        end
        
        
%#Overaal Control
    alpha = 90;
    a=90:0.5:180;
    B=(2-(2/180)*a+(1/pi)*sind(2*a));
    L_TCR = 517.59e-3;
    C = 3.135e-6;
    Xeq_TCR = 1.1199;
    Xeq_TSC = -5.8809; 
    %Xeq_TCR = 1.3596;
    Xeq_FC = -6.35137;
    
    f = 50;
    d = 15;
    Qdesired = (4*(Vdesired*cosd(d)-Vdesired^2))/2.066;

    FCTCR_Min = 0.7;
    FCTCR_Max = 1.056;
    FCTCR_TSC1_Min = 1.056;
    FCTCR_TSC1_Max = 1.165;
    FCTCR_TSC2_Min = 1.165;
    FCTCR_TSC2_Max = 1.3;


        if(Vdesired>=FCTCR_Min && Vdesired <= FCTCR_Max)
            FCTCR_EN = 1;
        else
            FCTCR_EN = 0;
        end
        if(Vdesired>FCTCR_TSC1_Min && Vdesired <= FCTCR_TSC1_Max)
            FCTCR_EN = 1;
            TSC1_EN = 1;
        else
            TSC1_EN = 0;
        end
        if(Vdesired>FCTCR_TSC2_Min && Vdesired <= FCTCR_TSC2_Max)||Vdesired > FCTCR_TSC2_Max
            FCTCR_EN = 1;
            TSC1_EN = 1;
            TSC2_EN = 1;

        else
            TSC2_EN = 0;
        end
        Qachievable = (Vdesired^2)* ((TSC1_EN/Xeq_TSC)+(TSC2_EN/Xeq_TSC)+(1/Xeq_FC));
        Qrequired = Qdesired - Qachievable;
        ILrequired = (Qrequired/Vdesired)/3;
        Iscaled = (ILrequired*3*Xeq_TCR/Vdesired);
        i=1;
        while i< 182
        if abs(Iscaled) < abs(B(1,i)) && abs(Iscaled) >= abs(B(1,i+1))
            alpha= a(1,i);
        end
        i=i+1;
        end
        triggerlevel = alpha*(0.5*mul/180);
        if Iscaled>1
            triggerlevel= 0.25;
        end
        if Vdesired > 1.29
             triggerlevel =.5;
        end

== matlab function SVC/SVC Control/TSC1/TSC_Control//phase b/TSC_Conrtrol ==
  data: v01 output; t1 output; t2 output; vc input; v1 input; v2 input; v0 input; flag output; flag1 input; en1 input; t10 input; vref input; wt input; wt_half output
function [v01,t1,t2,flag,wt_half] = TSC_control(vc,v1,v2,v0,flag1,en1,t10,vref,wt)
wt=wt/(2*pi);
if(wt>=0.5)
    wt_half = wt - 0.5;
else
    wt_half = wt;
end
flag =flag1;
v01=v0;
     t1=0;
     t2=0;

if en1==1
  
   if flag>1 
             

                if (t10==1)
                t1=1; t2=1;

                else 
                    t1=0;t2=0;
                end
         if vref>1.29
            t1=1;t2=1;
         end 


   elseif flag<1
        t1=0;
        t2=0;
        if abs(vc)< 1e-5 && abs(v0)<1e-2
             t2=1;
              t1=1;
                
                    flag=flag+.005;
        end
        if vc>=0 && v0>0
            if abs(v0-vc)<1e-3 || (v1 > v2 && v1>v0 && vc>v1)
                    t2=1;
                    t1=1;
                
                    flag=flag+.005;
            end
        end
        if vc<=0 && v0<0
            if abs(v0-vc)<1e-3|| (v1<v2 && v1<v0 && vc<v1)
                    t1=1;
                    t2=1;
                    flag=flag+.005;
            end
        end
  end
    
end
    
if en1==0
    flag=0;
end

== matlab function SVC/SVC Control/TSC1/TSC_Control//phase c/TSC_Conrtrol ==
  data: v01 output; t1 output; t2 output; vc input; v1 input; v2 input; v0 input; flag output; flag1 input; en1 input; t10 input; vref input; wt input; wt_half output

    
function [v01,t1,t2,flag,wt_half] = TSC_control(vc,v1,v2,v0,flag1,en1,t10,vref,wt)
wt=wt/(2*pi);
if(wt>=0.5)
    wt_half = wt - 0.5;
else
    wt_half = wt;
end
flag =flag1;
v01=v0;
     t1=0;
     t2=0;

if en1==1
  
   if flag>1 
             

                if (t10==1)
                t1=1; t2=1;

                else 
                    t1=0;t2=0;
                end
         if vref>1.29
            t1=1;t2=1;
         end 


   elseif flag<1
        t1=0;
        t2=0;
        if abs(vc)< 1e-5 && abs(v0)<1e-2
             t2=1;
              t1=1;
                
                    flag=flag+.005;
        end
        if vc>=0 && v0>0
            if abs(v0-vc)<1e-3 || (v1 > v2 && v1>v0 && vc>v1)
                    t2=1;
                    t1=1;
                
                    flag=flag+.005;
            end
        end
        if vc<=0 && v0<0
            if abs(v0-vc)<1e-3|| (v1<v2 && v1<v0 && vc<v1)
                    t1=1;
                    t2=1;
                    flag=flag+.005;
            end
        end
  end
    
end
    

if en1==0
    flag=0;
end
    

    
  if en1==0
    flag=0;
end

== matlab function SVC/SVC Control/TSC2/TSC_Control//phase a/TSC_Conrtrol ==
  data: v01 output; t1 output; t2 output; vc input; v1 input; v2 input; v0 input; flag output; flag1 input; en1 input; t10 input; vref input; wt input; wt_half output
function [v01,t1,t2,flag,wt_half] = TSC_control(vc,v1,v2,v0,flag1,en1,t10,vref,wt)
wt=wt/(2*pi);
if(wt>=0.5)
    wt_half = wt - 0.5;
else
    wt_half = wt;
end
flag =flag1;
v01=v0;
     t1=0;
     t2=0;

if en1==1
  
   if flag>1 
             

                if (t10==1)
                t1=1; t2=1;

                else 
                    t1=0;t2=0;
                end
         if vref>1.29
            t1=1;t2=1;
         end 


   elseif flag<1
        t1=0;
        t2=0;
        if abs(vc)< 1e-5 && abs(v0)<1e-2
             t2=1;
              t1=1;
                
                    flag=flag+.005;
        end
        if vc>=0 && v0>0
            if abs(v0-vc)<1e-3 || (v1 > v2 && v1>v0 && vc>v1)
                    t2=1;
                    t1=1;
                
                    flag=flag+.005;
            end
        end
        if vc<=0 && v0<0
            if abs(v0-vc)<1e-3|| (v1<v2 && v1<v0 && vc<v1)
                    t1=1;
                    t2=1;
                    flag=flag+.005;
            end
        end
  end
    
end
    


    if en1==0
    flag=0;
end

== matlab function SVC/SVC Control/TSC2/TSC_Control//phase b/TSC_Conrtrol ==
  data: v01 output; t1 output; t2 output; vc input; v1 input; v2 input; v0 input; flag output; flag1 input; en1 input; t10 input; vref input; wt input; wt_half output
function [v01,t1,t2,flag,wt_half] = TSC_control(vc,v1,v2,v0,flag1,en1,t10,vref,wt)
wt=wt/(2*pi);
if(wt>=0.5)
    wt_half = wt - 0.5;
else
    wt_half = wt;
end
flag =flag1;
v01=v0;
     t1=0;
     t2=0;

if en1==1
  
   if flag>1 
             

                if (t10==1)
                t1=1; t2=1;

                else 
                    t1=0;t2=0;
                end
         if vref>1.29
            t1=1;t2=1;
         end 


   elseif flag<1
        t1=0;
        t2=0;
        if abs(vc)< 1e-5 && abs(v0)<1e-2
             t2=1;
              t1=1;
                
                    flag=flag+.005;
        end
        if vc>=0 && v0>0
            if abs(v0-vc)<1e-3 || (v1 > v2 && v1>v0 && vc>v1)
                    t2=1;
                    t1=1;
                
                    flag=flag+.005;
            end
        end
        if vc<=0 && v0<0
            if abs(v0-vc)<1e-3|| (v1<v2 && v1<v0 && vc<v1)
                    t1=1;
                    t2=1;
                    flag=flag+.005;
            end
        end
  end
    
end
    
if en1==0
    flag=0;
end

== matlab function SVC/SVC Control/TSC2/TSC_Control//phase c/TSC_Conrtrol ==
  data: v01 output; t1 output; t2 output; vc input; v1 input; v2 input; v0 input; flag output; flag1 input; en1 input; t10 input; vref input; wt input; wt_half output
function [v01,t1,t2,flag,wt_half] = TSC_control(vc,v1,v2,v0,flag1,en1,t10,vref,wt)
wt=wt/(2*pi);
if(wt>=0.5)
    wt_half = wt - 0.5;
else
    wt_half = wt;
end
flag =flag1;
v01=v0;
     t1=0;
     t2=0;

if en1==1
  
   if flag>1 
             

                if (t10==1)
                t1=1; t2=1;

                else 
                    t1=0;t2=0;
                end
         if vref>1.29
            t1=1;t2=1;
         end 


   elseif flag<1
        t1=0;
        t2=0;
        if abs(vc)< 1e-5 && abs(v0)<1e-2
             t2=1;
              t1=1;
                
                    flag=flag+.005;
        end
        if vc>=0 && v0>0
            if abs(v0-vc)<1e-3 || (v1 > v2 && v1>v0 && vc>v1)
                    t2=1;
                    t1=1;
                
                    flag=flag+.005;
            end
        end
        if vc<=0 && v0<0
            if abs(v0-vc)<1e-3|| (v1<v2 && v1<v0 && vc<v1)
                    t1=1;
                    t2=1;
                    flag=flag+.005;
            end
        end
  end
    
end
    
if en1==0
    flag=0;
end
